simulink model "Arm_cobot"  (Simulink 8.3)
settings: Solver=ode1  StartTime=0.0  StopTime=inf  FixedStep=TA  RelTol=1e-3
PreLoadFcn:
  | startup
  | gui_starter
  | init_starter
PostLoadFcn:
  | init_check
InitFcn:
  | init_starter
undefined symbols (not defined in the file): alphaM, alphaT, Arm7ConLib, Arms2, baseOffset_x, baseOffset_y, baseOffset_z, betaM, betaT, cobotNa, cobotNb, D1, D2, D3, D4, D5, D6, D7, d_FTS_EE_L, d_FTS_EE_R, DD1, DD2, DD3, DD4, DD5, DD6, DD7, Do, Dp, EEL, EER, Fcal_L, Fcal_R, I1, I2, I3, I4, I5, I6, I7, IFL, IFR, impuls2rad_L, impuls2rad_R, Inert_L, Inert_R, KdC, KiC, Ko, Kp, KpC, LTool_L, LTool_R, mEE_L, mEE_R, Mo, Mp, P1, P2, P3 ... (+28)
libraries: sensoray x16, rtai_utilities x11, simulink x2, jr3lib x2, Interface x1
(part 1 of 3)
settings Model: Creator=mock  LastModifiedBy=wirnshofer  SimulationMode=external  ExtModeAutoUpdateStatusClock=off
settings DataIOCC: LimitDataPoints=off  SaveFormat=Structure
settings OptimizationCC: BlockReduction=off  BooleanDataType=off  ExpressionDepthLimit=2147483647  InitFltsAndDblsToZero=on
settings DebuggingCC: AlgebraicLoopMsg=none  SaveWithParameterizedLinksMsg=none  SignalResolutionControl=TryResolveAllWithWarning  SolverPrmCheckMsg=none  MultiTaskDSMMsg=warning  MultiTaskCondExecSysMsg=none  FcnCallInpInsideContextMsg=UseLocalSettings  UnconnectedInputMsg=none  UnconnectedOutputMsg=none  UnconnectedLineMsg=none  StrictBusMsg=None
settings HardwareCC: TargetHWDeviceType=32-bit Generic
settings SFSimCC: SimParseCustomCode=off
settings RTWCC: SystemTargetFile=prt.tlc  TemplateMakefile=prt.tmf  Description=Linux PREEMPT_RT Real-Time Target  ProcessScript=prt_make_rtw_hook  CustomLibrary=../../../../lib/libKinematicTypes.a ../../../../lib/libManipulation.a ../../../../lib/libkogmo_rtdb.a  IncludeERTFirstTime=on
settings RTWCC: CustomInclude=|
  | ../sfunctions/COMMON/InterfaceNew
  | ../sfunctions/COMMON/CollisionDetection
  | ../sfunctions/COMMON/PoseInterpolationNew
  | ../sfunctions/COMMON/PoseSpeedInterpolation
  | ../sfunctions/COMMON/Switching
  | ../sfunctions/COMMON/Helper
  | ../sfunctions/COMMON/Information
  | ../library/Animation
  | ../../../arch/rtdbobjects
  | ../../../arch
  | ../../../../opt/kogmo-rtdb/include
settings RTWCC: CustomSource=|
  | constant_information.cpp
  | ArmInterfaceNew.cpp
  | SwitchingX.cpp
  | Command_Classifier.cpp
  | PoseInterpolation_Code.cpp
  | PoseSpeedInterpolation_Code.cpp
  | armCDInterface.cpp
settings STFCustomTargetCC: TargetLangStandard=C99 (ISO)  CodeReplacementLibrary=GNU99 (GNU)  ModelReferenceCompliant=off  GeneratePreprocessorConditionals=Disable all  MatFileLogging=on  CPPClassGenCompliant=on  SystemTargetFile=prt.tlc
settings GRTTargetCC: TargetLangStandard=C99 (ISO)  CodeReplacementLibrary=GNU99 (GNU)  ModelReferenceCompliant=off  ParMdlRefBuildCompliant=off  CompOptLevelCompliant=off  ConcurrentExecutionCompliant=off  ExtModeMexArgs='cobot2a'

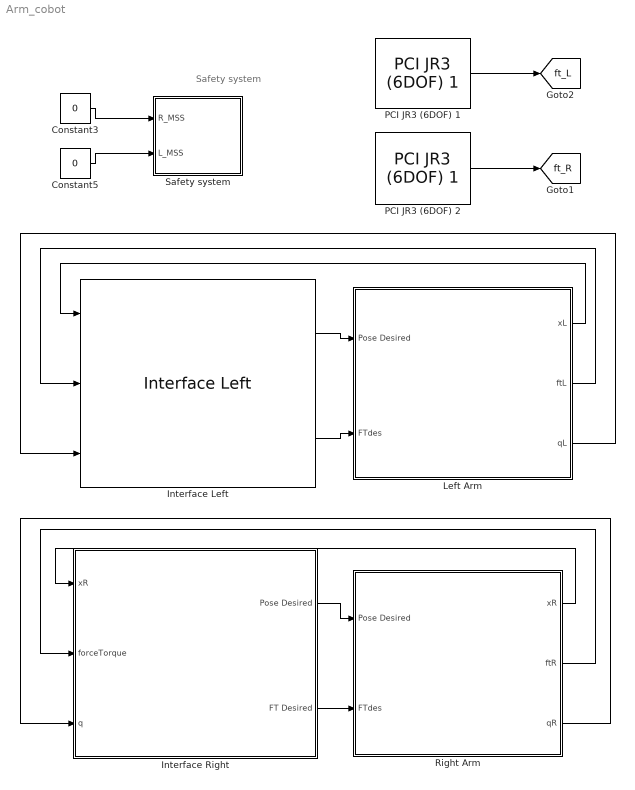
== system Arm_cobot ==
  note: Safety system
  Constant3 : Constant  Value=0
  Constant5 : Constant  Value=0
  Interface Left : Interface/Interface Left  SystemSampleTime=-1
  Interface Right : Subsystem  AncestorBlock=Interface/Interface Right  mask(Interface right){}
      settings: CopyFcn=inital_sources
      mask Display:
      | image(imread('Cobot_right.png'))
      | color('blue');
      | port_label('input',1, 'xR')
      | port_label('input',2, 'forceTorque')
      | port_label('input',3, 'q')
      | 
      | port_label('output',1, 'Pose Desired')
      | port_label('output',2, 'FT Desired')
  Left Arm : Subsystem  Priority=1
  PCI JR3 (6DOF) 1 : jr3lib/PCI JR3 (6DOF) 1  bd_number=0  filter_nr=1  sampletime=simget(bdroot,'FixedStep')  begin_reset=off
  PCI JR3 (6DOF) 2 : jr3lib/PCI JR3 (6DOF) 1  bd_number=1  filter_nr=1  sampletime=simget(bdroot,'FixedStep')  begin_reset=off
  Right Arm : Subsystem  Priority=1
  Safety system : Subsystem
      mask Display: image(imread('RTAIstop.bmp'))
  tag scope: ft_L=global, ft_R=global
  wires:
  Left Arm/2(ftL) -> Interface Left/2
  Right Arm/2(ftR) -> Interface Right/2(forceTorque)
  PCI JR3 (6DOF) 1/1 -> [ft_L]
  Constant3/1 -> Safety system/1(R_MSS)
  Constant5/1 -> Safety system/2(L_MSS)
  PCI JR3 (6DOF) 2/1 -> [ft_R]
  Interface Left/1 -> Left Arm/1(Pose Desired)
  Interface Right/1(Pose Desired) -> Right Arm/1(Pose Desired)
  Interface Left/2 -> Left Arm/2(FTdes)
  Left Arm/1(xL) -> Interface Left/1
  Left Arm/3(qL) -> Interface Left/3
  Interface Right/2(FT Desired) -> Right Arm/2(FTdes)
  Right Arm/1(xR) -> Interface Right/1(xR)
  Right Arm/3(qR) -> Interface Right/3(q)

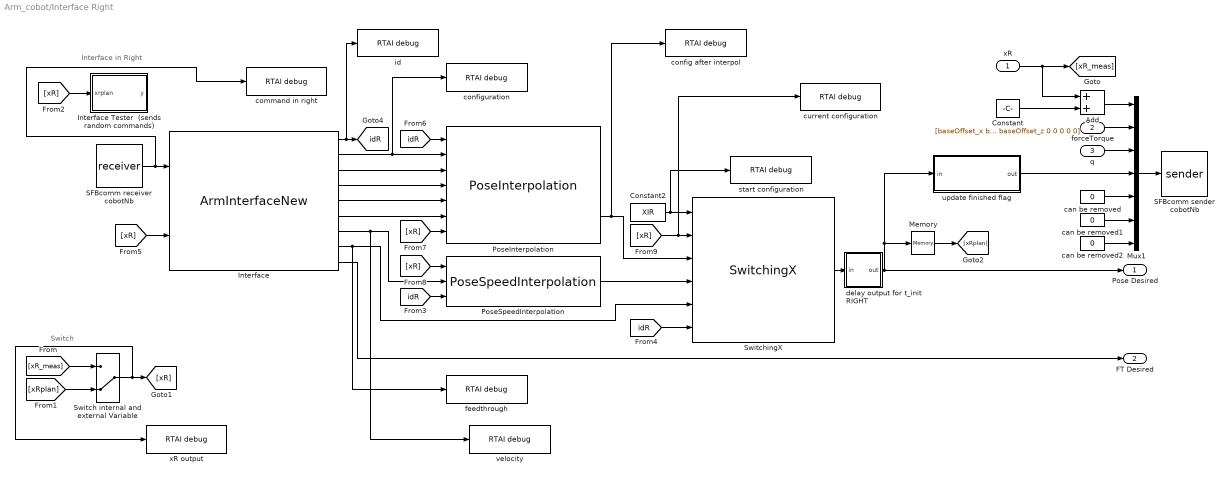
== system Arm_cobot/Interface Right ==
  note: Switch
  note: Interface in Right
  xR : Inport
  forceTorque : Inport  Port=2
  q : Inport  Port=3
  Add : Sum
  Constant : Constant  Value=[baseOffset_x baseOffset_y baseOffset_z 0 0 0 0 0]
  Constant2 : Constant  Value=XIR
  Interface : S-Function  FunctionName=ArmInterfaceNew  Parameters=xoffset,yoffset,zoffset  EnableBusSupport=off  mask{xoffset=baseOffset_x, yoffset=baseOffset_y, zoffset=baseOffset_z}
      mask prompts: xoffset "Base X Offset"; yoffset "Base Y Offset"; zoffset "Base Z Offset"
      mask Display:
      | port_label('input',1,'Command In')
      | port_label('input',2,'Configuration Current')
      | 
      | port_label('output',1,'CmdId')
      | port_label('output',2,'Configuration')
      | port_label('output',3,'Flags (replan/via)')
      | port_label('output',4,'Control Flow (count/total)')
      | port_label('output',5,'Time')
      | port_label('output',6,'Derivatives')
      | port_label('output',7,'Configuration Velocity')
      | port_label('output',8,'Feedthrough')
      | port_label('output',9,'FT')
  Interface Tester  (sends random commands) : MATLAB Function  TreatAsAtomicUnit=on
  Memory : Memory
  Mux1 : Mux  Inputs=7
  PoseInterpolation : S-Function  FunctionName=PoseInterpolation  EnableBusSupport=off
      mask Display:
      | port_label('input',1,'CmdId')
      | port_label('input',2,'Goal Configuration')
      | port_label('input',3,'Flags')
      | port_label('input',4,'Control Flow')
      | port_label('input',5,'Time')
      | port_label('input',6,'Derivatives')
      | port_label('input',7,'Current Configuration')
      | 
      | port_label('output',1,'Finish')
      | port_label('output',2,'Configuration')
  PoseSpeedInterpolation : S-Function  FunctionName=PoseSpeedInterpolation  EnableBusSupport=off
      mask Display:
      | port_label('input',1,'Current Configuration')
      | port_label('input',2,'Goal Configuration Speed')
      | port_label('input',3,'CmdId')
      | 
      | port_label('output',1,'Configuration')
  SFBcomm receiver cobotNb : S-Function  FunctionName=receiver  Parameters=localPort streamID remoteSettings portNames portWidths sampleTime outputLatency outputIdleTime connectTimeout  EnableBusSupport=off  mask(SFBcomm){localPort=8565, streamID=2, remoteSettings=[cobotNb ':8566'], portNames=A, portWidths=23, outputLatency=off, outputIdleTime=off, connectTimeout=200, sampleTime=TA}
      mask prompts: localPort "Local Port"; streamID "Stream ID"; remoteSettings "Remote Settings"; portNames "Port Names"; portWidths "Port Widths"; outputLatency "Output Latency"; outputIdleTime "Output Idle Time"; connectTimeout "Connect Timeout (in ms)"; sampleTime "Sample Time (-1 for inherited):"
      mask help: Receives data via SFB comm
      mask init:
      | idx=[0 strfind(portNames,' ') length(portNames)];
      | ddt=strfind(outputLatency,'on');
      | dit=strfind(outputIdleTime,'on');
      | 
      | for i=1:17
      |  if(i<length(idx))
      |   portnumber(i)=i;
      |   label{i}=portNames(idx(i)+1:idx(i+1));
      |  elseif((i==length(idx))&&(length(ddt)>0))
      |   portnumber(i)=i;
      |   label{i}='dt';
      |  elseif((i==length(idx))&&(length(dit)>0))
      |   portnumber(i)=i;
      |   label{i}='it';
      |  elseif((i==length(idx)+1)&&(length(ddt)>0)&&(length(dit)>0))
      |   portnumber(i)=i;
      |   label{i}='it';
      |  else
      |   portnumber(i)=1;
      |   label{i}=label{1};
      |  end
      | end
      mask Display:
      | image(imread('sfbcomm1.bmp'))
      | 
      | port_label('output',portnumber( 1),label{ 1})
      | port_label('output',portnumber( 2),label{ 2})
      | port_label('output',portnumber( 3),label{ 3})
      | port_label('output',portnumber( 4),label{ 4})
      | port_label('output',portnumber( 5),label{ 5})
      | port_label('output',portnumber( 6),label{ 6})
      | port_label('output',portnumber( 7),label{ 7})
      | port_label('output',portnumber( 8),label{ 8})
      | port_label('output',portnumber( 9),label{ 9})
      | port_label('output',portnumber(10),label{10})
      | port_label('output',portnumber(11),label{11})
      | port_label('output',portnumber(12),label{12})
      | port_label('output',portnumber(13),label{13})
      | port_label('output',portnumber(14),label{14})
      | port_label('output',portnumber(15),label{15})
      | port_label('output',portnumber(16),label{16})
      | port_label('output',portnumber(17),label{17})
  SFBcomm sender cobotNb : S-Function  FunctionName=sender  Parameters=localPort streamID remoteSettings portNames sampleTime connectTimeout  EnableBusSupport=off  mask(SFBcomm){localPort=8665, streamID=3, remoteSettings=[cobotNb ':8666'], portNames=A, connectTimeout=200, sampleTime=-1}
      mask prompts: localPort "Local Port"; streamID "Stream ID"; remoteSettings "Remote Settings"; portNames "Port Names"; connectTimeout "Connect Timeout (in ms)"; sampleTime "Sample time (-1 for inherited):"
      mask help: Sends data via SFB comm
      mask init:
      | idx=[0 strfind(portNames,' ') length(portNames)];
      | 
      | for i=1:16
      |  if(i<length(idx))
      |   portnumber(i)=i;
      |   label{i}=portNames(idx(i)+1:idx(i+1));
      |  else
      |   portnumber(i)=1;
      |   label{i}=label{1};
      |  end
      | end
      mask Display:
      | image(imread('sfbcomm1.bmp'))
      | port_label('input',portnumber( 1),label{ 1})
      | port_label('input',portnumber( 2),label{ 2})
      | port_label('input',portnumber( 3),label{ 3})
      | port_label('input',portnumber( 4),label{ 4})
      | port_label('input',portnumber( 5),label{ 5})
      | port_label('input',portnumber( 6),label{ 6})
      | port_label('input',portnumber( 7),label{ 7})
      | port_label('input',portnumber( 8),label{ 8})
      | port_label('input',portnumber( 9),label{ 9})
      | port_label('input',portnumber(10),label{10})
      | port_label('input',portnumber(11),label{11})
      | port_label('input',portnumber(12),label{12})
      | port_label('input',portnumber(13),label{13})
      | port_label('input',portnumber(14),label{14})
      | port_label('input',portnumber(15),label{15})
      | port_label('input',portnumber(16),label{16})
  Switch internal and external Variable : ManualSwitch  CurrentSetting=0
  SwitchingX : S-Function  FunctionName=SwitchingX  EnableBusSupport=off
      mask Display:
      | port_label('input',1,'Start Configuration')
      | port_label('input',2,'Current Configuration')
      | port_label('input',3,'Config from PoseInter')
      | port_label('input',4,'Config from SpeedInter')
      | port_label('input',5,'Config from Feedtrough')
      | port_label('input',6,'CmdId')
      | 
      | port_label('output',1,'Configuration')
  can be removed : Constant  Value=0
  can be removed1 : Constant  Value=0
  can be removed2 : Constant  Value=0
  command in right : rtai_utilities/RTAI debug  rate=1
  config after interpol : rtai_utilities/RTAI debug  rate=1
  configuration : rtai_utilities/RTAI debug  rate=1
  current configuration : rtai_utilities/RTAI debug  rate=1
  delay output for t_init RIGHT : Subsystem
  feedthrough : rtai_utilities/RTAI debug  rate=1
  id : rtai_utilities/RTAI debug  rate=1
  start configuration : rtai_utilities/RTAI debug  rate=1
  update finished flag : MATLAB Function  TreatAsAtomicUnit=on
  velocity : rtai_utilities/RTAI debug  rate=1
  xR output : rtai_utilities/RTAI debug  rate=1
  Pose Desired : Outport
  FT Desired : Outport  Port=2
  tag scope: idR=global
  wires:
  Switch internal and external Variable/1 -> xR output/1, [xR]
  [xRplan] -> Switch internal and external Variable/2
  Memory/1 -> [xRplan]
  [xR_meas] -> Switch internal and external Variable/1
  xR/1 -> [xR_meas], Add/1
  Constant2/1 -> start configuration/1, SwitchingX/1
  [xR] -> current configuration/1, SwitchingX/2
  PoseInterpolation/2 -> config after interpol/1, SwitchingX/3
  PoseSpeedInterpolation/1 -> SwitchingX/4
  Interface/8 -> feedthrough/1, SwitchingX/5
  [idR] -> SwitchingX/6
  [xR] -> Interface/2
  [xR] -> PoseSpeedInterpolation/1
  [xR] -> PoseInterpolation/7
  SFBcomm receiver cobotNb/1 -> command in right/1, Interface/1
  [xR] -> Interface Tester  (sends random commands)/1(xrplan)
  Interface/9 -> FT Desired/1
  update finished flag/1(out) -> Mux1/4
  [idR] -> PoseInterpolation/1
  Interface/6 -> PoseInterpolation/6
  Interface/5 -> PoseInterpolation/5
  delay output for t_init RIGHT/1(out) -> Memory/1, update finished flag/1(in), Pose Desired/1
  Interface/7 -> velocity/1, PoseSpeedInterpolation/2
  [idR] -> PoseSpeedInterpolation/3
  Interface/1 -> id/1, [idR]
  SwitchingX/1 -> delay output for t_init RIGHT/1(in)
  can be removed2/1 -> Mux1/7
  can be removed1/1 -> Mux1/6
  can be removed/1 -> Mux1/5
  Constant/1 -> Add/2
  Add/1 -> Mux1/1
  Mux1/1 -> SFBcomm sender cobotNb/1
  q/1 -> Mux1/3
  forceTorque/1 -> Mux1/2
  Interface/4 -> PoseInterpolation/4
  Interface/3 -> PoseInterpolation/3
  Interface/2 -> configuration/1, PoseInterpolation/2

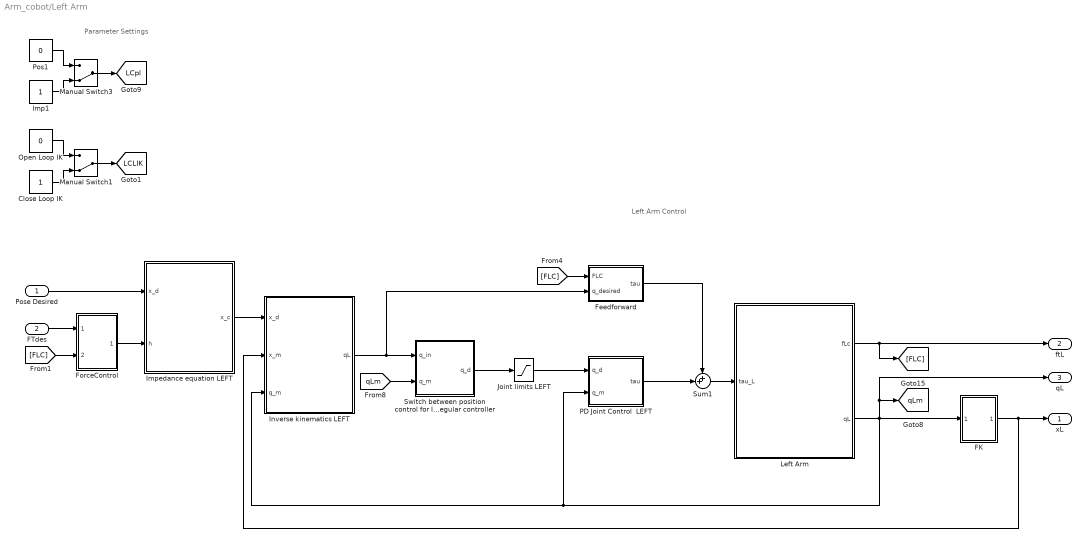
== system Arm_cobot/Left Arm ==
  note: Parameter Settings
  note: Left Arm Control
  Pose Desired : Inport
  FTdes : Inport  Port=2
  Close Loop IK : Constant
  FK : Subsystem
  Feedforward : Subsystem
  ForceControl : Subsystem
  Imp1 : Constant
  Impedance equation LEFT : Subsystem
  Inverse kinematics LEFT : Subsystem
  Joint limits LEFT : Saturate  UpperLimit=q_maxL  LowerLimit=q_minL
  Left Arm : Subsystem
  Manual Switch1 : ManualSwitch  Priority=1  CurrentSetting=0
  Manual Switch3 : ManualSwitch  Priority=1  CurrentSetting=0
  Open Loop IK : Constant  Value=0
  PD Joint Control  LEFT : Subsystem  AncestorBlock=Arm7lib/PD Joint
  Pos1 : Constant  Value=0
  Sum1 : Sum  Inputs=++|
  Switch between position control for Init position and regular controller : Subsystem
  xL : Outport
  ftL : Outport  Port=2
  qL : Outport  Port=3
  tag scope: LCLIK=global, LCpl=global, qLm=global
  wires:
  Left Arm/2(qL) -> FK/1(q_m), PD Joint Control  LEFT/2(q_m), Inverse kinematics LEFT/3(q_m), qL/1, [qLm]
  Left Arm/1(fLc) -> ftL/1, [FLC]
  [qLm] -> Switch between position control for Init position and regular controller/2(q_m)
  Joint limits LEFT/1 -> PD Joint Control  LEFT/1(q_d)
  Imp1/1 -> Manual Switch3/2
  Pos1/1 -> Manual Switch3/1
  Manual Switch3/1 -> [LCpl]
  Switch between position control for Init position and regular controller/1(q_d) -> Joint limits LEFT/1
  Pose Desired/1 -> Impedance equation LEFT/1(x_d)
  FK/1(pose) -> xL/1, Inverse kinematics LEFT/2(x_m)
  Inverse kinematics LEFT/1(qL) -> Switch between position control for Init position and regular controller/1(q_in), Feedforward/2(q_desired)
  Close Loop IK/1 -> Manual Switch1/2
  Open Loop IK/1 -> Manual Switch1/1
  Manual Switch1/1 -> [LCLIK]
  ForceControl/1(Out1) -> Impedance equation LEFT/2(h)
  [FLC] -> ForceControl/2(FTmesL)
  FTdes/1 -> ForceControl/1(FTdesLeft)
  Sum1/1 -> Left Arm/1(tau_L)
  PD Joint Control  LEFT/1(tau) -> Sum1/2
  Impedance equation LEFT/1(x_c) -> Inverse kinematics LEFT/1(x_d)
  [FLC] -> Feedforward/1(FLC)
  Feedforward/1(tau) -> Sum1/1

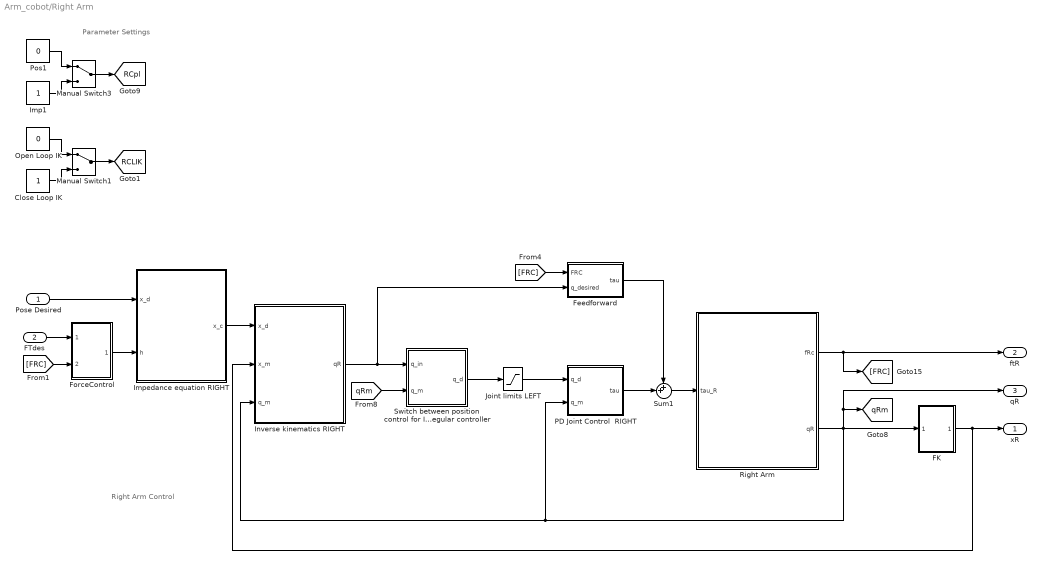
== system Arm_cobot/Right Arm ==
  note: Parameter Settings
  note: Right Arm Control
  Pose Desired : Inport
  FTdes : Inport  Port=2
  Close Loop IK : Constant
  FK : Subsystem
  Feedforward : Subsystem
  ForceControl : Subsystem
  Imp1 : Constant
  Impedance equation RIGHT : Subsystem
  Inverse kinematics RIGHT : Subsystem
  Joint limits LEFT : Saturate  UpperLimit=q_maxR  LowerLimit=q_minR
  Manual Switch1 : ManualSwitch
  Manual Switch3 : ManualSwitch
  Open Loop IK : Constant  Value=0
  PD Joint Control  RIGHT : Subsystem  AncestorBlock=Arm7lib/PD Joint
  Pos1 : Constant  Value=0
  Right Arm : Subsystem
  Sum1 : Sum  Inputs=++|
  Switch between position control for Init position and regular controller : Subsystem
  xR : Outport
  ftR : Outport  Port=2
  qR : Outport  Port=3
  tag scope: RCLIK=global, RCpl=global, qRm=global
  wires:
  Right Arm/2(qR) -> FK/1(q_m), PD Joint Control  RIGHT/2(q_m), Inverse kinematics RIGHT/3(q_m), qR/1, [qRm]
  Right Arm/1(fRc) -> ftR/1, [FRC]
  [qRm] -> Switch between position control for Init position and regular controller/2(q_m)
  Joint limits LEFT/1 -> PD Joint Control  RIGHT/1(q_d)
  Imp1/1 -> Manual Switch3/2
  Pos1/1 -> Manual Switch3/1
  Manual Switch3/1 -> [RCpl]
  Switch between position control for Init position and regular controller/1(q_d) -> Joint limits LEFT/1
  Sum1/1 -> Right Arm/1(tau_R)
  Pose Desired/1 -> Impedance equation RIGHT/1(x_d)
  FK/1(pose) -> xR/1, Inverse kinematics RIGHT/2(x_m)
  Inverse kinematics RIGHT/1(qR) -> Switch between position control for Init position and regular controller/1(q_in), Feedforward/2(q_desired)
  Close Loop IK/1 -> Manual Switch1/2
  Open Loop IK/1 -> Manual Switch1/1
  Manual Switch1/1 -> [RCLIK]
  [FRC] -> Feedforward/1(FRC)
  FTdes/1 -> ForceControl/1(FTdesRight)
  [FRC] -> ForceControl/2(FTmesR)
  ForceControl/1(Out1) -> Impedance equation RIGHT/2(h)
  Impedance equation RIGHT/1(x_c) -> Inverse kinematics RIGHT/1(x_d)
  PD Joint Control  RIGHT/1(tau) -> Sum1/2
  Feedforward/1(tau) -> Sum1/1

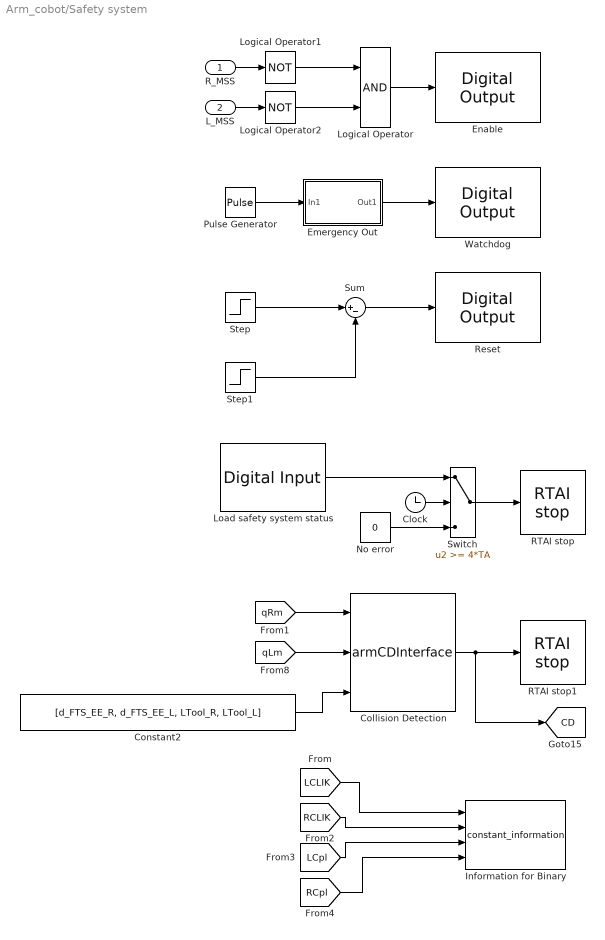
== system Arm_cobot/Safety system ==
  R_MSS : Inport
  L_MSS : Inport  Port=2
  Clock : Clock
  Collision Detection : S-Function  FunctionName=armCDInterface  EnableBusSupport=off
  Constant2 : Constant  Value=[d_FTS_EE_R, d_FTS_EE_L, LTool_R, LTool_L]
  Emergency Out : Subsystem
  Enable : sensoray/Digital Output  BoardNumber=0  Channels=27  InitialOutputs=0  FinalOutputs=0  SampleTime=-1
  Information for Binary : S-Function  Priority=2  FunctionName=constant_information  Parameters="cobotNa, EEL, EER,  get_param('Arm_cobot/Interface Left/Switch internal and external Variable', 'sw'), get_param('Arm_cobot/Interface Right/Switch internal and external Variable', 'sw')"  EnableBusSupport=off
  Load safety system status : sensoray/Digital Input  BoardNumber=0  Channels=25  SampleTime=simget(bdroot,'FixedStep')
  Logical Operator : Logic  AllPortsSameDT=off
  Logical Operator1 : Logic  Operator=NOT  AllPortsSameDT=off  OutDataTypeStr=boolean
  Logical Operator2 : Logic  Operator=NOT  AllPortsSameDT=off  OutDataTypeStr=boolean
  No error : Constant  Value=0
  Pulse Generator : DiscretePulseGenerator  PulseType=Time based  Period=2*TA  PulseWidth=50
  RTAI stop : rtai_utilities/RTAI stop
  RTAI stop1 : rtai_utilities/RTAI stop
  Reset : sensoray/Digital Output  BoardNumber=0  Channels=24  InitialOutputs=0  FinalOutputs=0  SampleTime=-1
  Step : Step  Time=0
  Step1 : Step  Time=2*TA
  Sum : Sum  Inputs=|+-  SaturateOnIntegerOverflow=on  InputSameDT=on  OutDataTypeStr=Inherit: Same as first input
  Switch : Switch  Threshold=4*TA  SaturateOnIntegerOverflow=on  InputSameDT=on
  Watchdog : sensoray/Digital Output  BoardNumber=0  Channels=26  InitialOutputs=0  FinalOutputs=0  SampleTime=-1
  tag scope: CD=global
  wires:
  Pulse Generator/1 -> Emergency Out/1(In1)
  Step/1 -> Sum/1
  Sum/1 -> Reset/1
  Step1/1 -> Sum/2
  Logical Operator/1 -> Enable/1
  R_MSS/1 -> Logical Operator1/1
  L_MSS/1 -> Logical Operator2/1
  Logical Operator1/1 -> Logical Operator/1
  Logical Operator2/1 -> Logical Operator/2
  Switch/1 -> RTAI stop/1
  Clock/1 -> Switch/2
  Load safety system status/1 -> Switch/1
  No error/1 -> Switch/3
  Collision Detection/1 -> RTAI stop1/1, [CD]
  [qLm] -> Collision Detection/2
  [qRm] -> Collision Detection/1
  Constant2/1 -> Collision Detection/3
  Emergency Out/1(Out1) -> Watchdog/1
  [LCLIK] -> Information for Binary/1
  [LCpl] -> Information for Binary/3
  [RCpl] -> Information for Binary/4
  [RCLIK] -> Information for Binary/2

== system Arm_cobot/Interface Right/delay output for t_init RIGHT ==
  in : Inport
  Clock : Clock
  Constant1 : Constant  Value=XIR
  Switch2 : Switch  Threshold=t_init  SaturateOnIntegerOverflow=on  InputSameDT=on
  out : Outport
  wires:
  Switch2/1 -> out/1
  in/1 -> Switch2/1
  Constant1/1 -> Switch2/3
  Clock/1 -> Switch2/2

== system Arm_cobot/Left Arm/FK ==
  q_m : Inport
  Constant1 : Constant  Value=LTool_L
  Demux : Demux  Outputs=[3 9 1]
  FK_L : S-Function  FunctionName=fk_l_S  EnableBusSupport=off
  Mux : Mux  Inputs=2
  Mux1 : Mux  Inputs=3
  Reshape : Reshape  OutputDimensionality=Customize  OutputDimensions=[3,3]
  S-Function1 : S-Function  FunctionName=rot2Q_S  EnableBusSupport=off
  pose : Outport
  wires:
  Constant1/1 -> Mux/1
  Mux/1 -> FK_L/1
  FK_L/1 -> Demux/1
  Demux/1 -> Mux1/1
  Demux/3 -> Mux1/3
  q_m/1 -> Mux/2
  Mux1/1 -> pose/1
  Reshape/1 -> S-Function1/1
  Demux/2 -> Reshape/1
  S-Function1/1 -> Mux1/2

== system Arm_cobot/Left Arm/Feedforward ==
  FLC : Inport
  q_desired : Inport  Port=2
  Constant1 : Constant  Value=[0 0 0 0 0 0]
  Constant2 : Constant  Value=[Inert_L, d_FTS_EE_L, mEE_L, p_EE_o_L]
  Demux : Demux  Outputs=[3,3]
  Derivative : Derivative
  Gain : Gain  Gain=-1
  Mux2 : Mux  Inputs=6
  S-Function : S-Function  FunctionName=dynmod_l_S  EnableBusSupport=off
  second  derivative : Subsystem  AncestorBlock=Arm7lib/PD Joint
  tau : Outport
  wires:
  q_desired/1 -> Mux2/3, Derivative/1, second  derivative/1(q)
  Mux2/1 -> S-Function/1
  S-Function/1 -> tau/1
  Constant2/1 -> Mux2/1
  Derivative/1 -> Mux2/5
  Demux/1 -> Mux2/2
  Demux/2 -> Mux2/4
  Gain/1 -> Demux/1
  Constant1/1 -> Gain/1
  second  derivative/1(qDotDot) -> Mux2/6

== system Arm_cobot/Left Arm/ForceControl ==
  FTdesLeft : Inport
  FTmesL : Inport  Port=2
  Abs : Abs
  Subsystem : Subsystem  mask{PF=PFL, IF=IFL, SF=SFL}
      mask prompts: PF "Proportional Gain"; IF "Integral Gain"; SF "Saturation"
      mask Display: disp('PI6')
  Sum : Sum  Inputs=|++
  Sum of Elements : Sum  Inputs=+
  Switch : Switch  Criteria=u2 ~= 0  Threshold=0.5
  lowpass : Subsystem
  Out1 : Outport
  wires:
  Sum/1 -> Subsystem/1(In1)
  Subsystem/1(Out1) -> Switch/1
  FTdesLeft/1 -> Sum/2, Abs/1
  Abs/1 -> Sum of Elements/1
  Sum of Elements/1 -> Subsystem/2(reset), Switch/2
  FTmesL/1 -> lowpass/1(fLc), Switch/3
  Switch/1 -> Out1/1
  lowpass/1(smoothed) -> Sum/1

== system Arm_cobot/Left Arm/Impedance equation LEFT ==
  x_d : Inport
  h : Inport  Port=2
  Constant1 : Constant  Value=zeros(1,7)
  Impedance  Equation : Subsystem  AncestorBlock="Arm7ConLib/Impedance  Equation"  mask{M_p=Mp, D_p=Dp, K_p=Kp, M_o=Mo, D_o=Do, K_o=Ko}
      mask prompts: M_p "Virtual mass (Translational)"; D_p "Damping matrix (translational)"; K_p "Stiffness matrix (translational)"; M_o "Virtual mass (rotational)"; D_o "Damping matrix (rotational)"; K_o "Stiffness matrix (rotational)"
  Switch : Switch  Threshold=0.5
  x_c : Outport
  wires:
  Constant1/1 -> Impedance  Equation/3(ddx_d), Impedance  Equation/2(dx_d)
  h/1 -> Impedance  Equation/4(h)
  x_d/1 -> Impedance  Equation/1(x_d), Switch/3
  Switch/1 -> x_c/1
  [LCpl] -> Switch/2
  Impedance  Equation/1(x_c) -> Switch/1

== system Arm_cobot/Left Arm/Inverse kinematics LEFT ==
  x_d : Inport
  x_m : Inport  Port=2
  q_m : Inport  Port=3
  IK_L weighted damped least square : Subsystem
  Pos1 : Constant  Value=zeros(7,1)
  Switch : Switch  Threshold=0.5
  pose error in task space : Subsystem
  qL : Outport
  wires:
  x_d/1 -> IK_L weighted damped least square/1(XL), pose error in task space/1(x_d)
  x_m/1 -> pose error in task space/2(x_m)
  IK_L weighted damped least square/1(q_damp) -> qL/1, IK_L weighted damped least square/2(qL)
  q_m/1 -> pose error in task space/3(qL)
  [LCLIK] -> Switch/2
  Switch/1 -> IK_L weighted damped least square/3(X_error)
  pose error in task space/1(X_error) -> Switch/1
  Pos1/1 -> Switch/3

== system Arm_cobot/Left Arm/Left Arm ==
  tau_L : Inport
  Arms : Subsystem  AncestorBlock=Arm7ConLib/Arms2
  fLc : Outport
  qL : Outport  Port=2
  wires:
  Arms/1(q _L) -> qL/1
  Arms/3(fLc) -> fLc/1
  tau_L/1 -> Arms/1(tau_L)

== system Arm_cobot/Left Arm/PD Joint Control  LEFT ==
  q_d : Inport
  q_m : Inport  Port=2
  PID Digital Derivative1 : Subsystem  mask(7 DOF PID Controller){P=[P1 P2 P3 P4 P5 P6 P7], I=[I1 I2 I3 I4 I5 I6 I7], D=[D1 D2 D3 D4 D5 D6 D7], N=[DD1 DD2 DD3 DD4 DD5 DD6 DD7]}
      mask prompts: P "Proportional:"; I "Integral"; D "Derivative:"; N "Derivative Divisor:"
      mask Display: disp('PID7')
  Sum1 : Sum  Inputs=-+|  SaturateOnIntegerOverflow=on  InputSameDT=on  OutDataTypeStr=Inherit: Same as first input
  tau : Outport
  wires:
  q_d/1 -> Sum1/2
  q_m/1 -> Sum1/1
  Sum1/1 -> PID Digital Derivative1/1(In1)
  PID Digital Derivative1/1(Out1) -> tau/1

== system Arm_cobot/Left Arm/Switch between position control for Init position and regular controller ==
  q_in : Inport
  q_m : Inport  Port=2
  BackToInit1 : Subsystem
  Clock : Clock
  Switch2 : Switch  Threshold=t_init  SaturateOnIntegerOverflow=on  InputSameDT=on
  q_d : Outport
  wires:
  q_in/1 -> Switch2/1
  Clock/1 -> Switch2/2
  BackToInit1/1(q [rad]) -> Switch2/3
  q_m/1 -> BackToInit1/1(JointAngles [rad])
  Switch2/1 -> q_d/1

== system Arm_cobot/Right Arm/FK ==
  q_m : Inport
  Constant1 : Constant  Value=LTool_R
  Demux : Demux  Outputs=[3 9 1]
  FK_R : S-Function  FunctionName=fk_r_S  EnableBusSupport=off
  Mux : Mux  Inputs=2
  Mux1 : Mux  Inputs=3
  Reshape : Reshape  OutputDimensionality=Customize  OutputDimensions=[3,3]
  S-Function1 : S-Function  FunctionName=rot2Q_S  EnableBusSupport=off
  pose : Outport
  wires:
  Constant1/1 -> Mux/1
  Mux/1 -> FK_R/1
  FK_R/1 -> Demux/1
  Demux/1 -> Mux1/1
  Demux/3 -> Mux1/3
  q_m/1 -> Mux/2
  Mux1/1 -> pose/1
  Reshape/1 -> S-Function1/1
  Demux/2 -> Reshape/1
  S-Function1/1 -> Mux1/2

== system Arm_cobot/Right Arm/Feedforward ==
  FRC : Inport
  q_desired : Inport  Port=2
  Constant1 : Constant  Value=[0 0 0 0 0 0]
  Constant2 : Constant  Value=[Inert_R, d_FTS_EE_R, mEE_R, p_EE_o_R]
  Demux : Demux  Outputs=[3,3]
  Derivative : Derivative
  Gain : Gain  Gain=-1
  Mux2 : Mux  Inputs=6
  S-Function : S-Function  FunctionName=dynmod_r_S  EnableBusSupport=off
  second  derivative : Subsystem  AncestorBlock=Arm7lib/PD Joint
  tau : Outport
  wires:
  q_desired/1 -> Mux2/3, Derivative/1, second  derivative/1(q)
  Mux2/1 -> S-Function/1
  S-Function/1 -> tau/1
  Constant2/1 -> Mux2/1
  Derivative/1 -> Mux2/5
  Demux/1 -> Mux2/2
  Demux/2 -> Mux2/4
  Gain/1 -> Demux/1
  Constant1/1 -> Gain/1
  second  derivative/1(qDotDot) -> Mux2/6

== system Arm_cobot/Right Arm/ForceControl ==
  FTdesRight : Inport
  FTmesR : Inport  Port=2
  Abs : Abs
  Subsystem : Subsystem  mask{PF=PFR, IF=IFR, SF=SFR}
      mask prompts: PF "Proportional Gain"; IF "Integral Gain"; SF "Saturation"
      mask Display: disp('PI6')
  Sum : Sum  Inputs=|++
  Sum of Elements : Sum  Inputs=+
  Switch : Switch  Criteria=u2 ~= 0  Threshold=0.5
  lowpass : Subsystem
  Out1 : Outport
  wires:
  Sum/1 -> Subsystem/1(In1)
  Subsystem/1(Out1) -> Switch/1
  FTdesRight/1 -> Sum/2, Abs/1
  Abs/1 -> Sum of Elements/1
  Sum of Elements/1 -> Subsystem/2(reset), Switch/2
  FTmesR/1 -> lowpass/1(fLc), Switch/3
  Switch/1 -> Out1/1
  lowpass/1(smoothed) -> Sum/1

== system Arm_cobot/Right Arm/Impedance equation RIGHT ==
  x_d : Inport
  h : Inport  Port=2
  Constant1 : Constant  Value=zeros(1,7)
  Impedance  Equation : Subsystem  AncestorBlock="Arm7ConLib/Impedance  Equation"  mask{M_p=Mp, D_p=Dp, K_p=Kp, M_o=Mo, D_o=Do, K_o=Ko}
      mask prompts: M_p "Virtual mass (Translational)"; D_p "Damping matrix (translational)"; K_p "Stiffness matrix (translational)"; M_o "Virtual mass (rotational)"; D_o "Damping matrix (rotational)"; K_o "Stiffness matrix (rotational)"
  Switch : Switch  Threshold=0.5
  x_c : Outport
  wires:
  Constant1/1 -> Impedance  Equation/3(ddx_d), Impedance  Equation/2(dx_d)
  Impedance  Equation/1(x_c) -> Switch/1
  h/1 -> Impedance  Equation/4(h)
  x_d/1 -> Impedance  Equation/1(x_d), Switch/3
  Switch/1 -> x_c/1
  [RCpl] -> Switch/2

== system Arm_cobot/Right Arm/Inverse kinematics RIGHT ==
  x_d : Inport
  x_m : Inport  Port=2
  q_m : Inport  Port=3
  IK_R weighted damped least square : Subsystem
  Switch : Switch  Threshold=0.5
  pose error in task space : Subsystem
  zeros : Constant  Value=zeros(7,1)
  qR : Outport
  wires:
  x_d/1 -> IK_R weighted damped least square/1(XR), pose error in task space/1(x_d)
  x_m/1 -> pose error in task space/2(x_m)
  IK_R weighted damped least square/1(q_damp) -> IK_R weighted damped least square/2(qR), qR/1
  q_m/1 -> pose error in task space/3(qR)
  [RCLIK] -> Switch/2
  Switch/1 -> IK_R weighted damped least square/3(X_error)
  pose error in task space/1(X_error) -> Switch/1
  zeros/1 -> Switch/3

== system Arm_cobot/Right Arm/PD Joint Control  RIGHT ==
  q_d : Inport
  q_m : Inport  Port=2
  PID Digital Derivative1 : Subsystem  mask(7 DOF PID Controller){P=[P1 P2 P3 P4 P5 P6 P7], I=[I1 I2 I3 I4 I5 I6 I7], D=[D1 D2 D3 D4 D5 D6 D7], N=[DD1 DD2 DD3 DD4 DD5 DD6 DD7]}
      mask prompts: P "Proportional:"; I "Integral"; D "Derivative:"; N "Derivative Divisor:"
      mask Display: disp('PID7')
  Sum1 : Sum  Inputs=-+|  SaturateOnIntegerOverflow=on  InputSameDT=on  OutDataTypeStr=Inherit: Same as first input
  tau : Outport
  wires:
  q_d/1 -> Sum1/2
  q_m/1 -> Sum1/1
  Sum1/1 -> PID Digital Derivative1/1(In1)
  PID Digital Derivative1/1(Out1) -> tau/1

== system Arm_cobot/Right Arm/Right Arm ==
  tau_R : Inport
  Arms : Subsystem  AncestorBlock=Arm7ConLib/Arms2
  fRc : Outport
  qR : Outport  Port=2
  wires:
  Arms/1(q _R) -> qR/1
  Arms/3(fRc) -> fRc/1
  tau_R/1 -> Arms/1(tau_R)

== system Arm_cobot/Right Arm/Switch between position control for Init position and regular controller ==
  q_in : Inport
  q_m : Inport  Port=2
  BackToInit1 : Subsystem
  Clock : Clock
  Switch2 : Switch  Threshold=t_init  SaturateOnIntegerOverflow=on  InputSameDT=on
  q_d : Outport
  wires:
  q_in/1 -> Switch2/1
  Clock/1 -> Switch2/2
  BackToInit1/1(q [rad]) -> Switch2/3
  q_m/1 -> BackToInit1/1(JointAngles [rad])
  Switch2/1 -> q_d/1

== system Arm_cobot/Safety system/Emergency Out ==
  In1 : Inport
  Fcn : Fcn  Expr=-u[1]+1
  Product : Product  RndMeth=Zero
  Out1 : Outport
  wires:
  [CD] -> Fcn/1
  In1/1 -> Product/2
  Product/1 -> Out1/1
  Fcn/1 -> Product/1

== system Arm_cobot/Left Arm/Feedforward/second  derivative ==
  q : Inport
  2ndDerivative3Points : MATLAB Function  TreatAsAtomicUnit=on
  Constant : Constant  Value=10*ones(1,7)
  Constant1 : Constant  Value=-10*ones(1,7)
  Memory : Memory
  Memory1 : Memory
  Rate Limiter Dynamic : simulink/Discontinuities/Rate Limiter Dynamic
  qDotDot : Outport
  wires:
  q/1 -> Memory/1, 2ndDerivative3Points/1(u0)
  Memory/1 -> Memory1/1, 2ndDerivative3Points/2(u1)
  Memory1/1 -> 2ndDerivative3Points/3(u2)
  Constant/1 -> Rate Limiter Dynamic/1
  Constant1/1 -> Rate Limiter Dynamic/3
  Rate Limiter Dynamic/1 -> qDotDot/1
  2ndDerivative3Points/1(y) -> Rate Limiter Dynamic/2

== system Arm_cobot/Left Arm/ForceControl/Subsystem ==
  In1 : Inport
  reset : Inport  Port=2
  Demux : Demux  Outputs=6
  Mux : Mux  Inputs=6
  PII : Subsystem  AncestorBlock=|  mask(PID(2) Controller){P=PF(1), I=IF(1), S=SF(1)}
      | Arm7lib/PID
      | Digital Derivative/PID +
      | digital Derivative2
      mask prompts: P "Proportional:"; I "Integral:"; S "Saturation:"
      mask help:
      | Enter Proportional(P), Integral(I), and Derivative(D) and divisor (N) terms.
      | P+I/s+Ds/(1/Ns+1)
      mask Help: This block implements a PID controller where parameters are entered for the Proportional, Integral and Derivative and divisor terms. Unmask this block to see how it works. The derivative term is implemented using an s/(s/N +1)  transfer function block. Making N large can create a "stiff" system.
      mask Display: disp('PI')
  PII1 : Subsystem  AncestorBlock=|  mask(PID(2) Controller){P=PF(2), I=IF(2), S=SF(2)}
      | Arm7lib/PID
      | Digital Derivative/PID +
      | digital Derivative2
      mask prompts: P "Proportional:"; I "Integral:"; S "Saturation:"
      mask help:
      | Enter Proportional(P), Integral(I), and Derivative(D) and divisor (N) terms.
      | P+I/s+Ds/(1/Ns+1)
      mask Help: This block implements a PID controller where parameters are entered for the Proportional, Integral and Derivative and divisor terms. Unmask this block to see how it works. The derivative term is implemented using an s/(s/N +1)  transfer function block. Making N large can create a "stiff" system.
      mask Display: disp('PI')
  PII2 : Subsystem  AncestorBlock=|  mask(PID(2) Controller){P=PF(3), I=IF(3), S=SF(3)}
      | Arm7lib/PID
      | Digital Derivative/PID +
      | digital Derivative2
      mask prompts: P "Proportional:"; I "Integral:"; S "Saturation:"
      mask help:
      | Enter Proportional(P), Integral(I), and Derivative(D) and divisor (N) terms.
      | P+I/s+Ds/(1/Ns+1)
      mask Help: This block implements a PID controller where parameters are entered for the Proportional, Integral and Derivative and divisor terms. Unmask this block to see how it works. The derivative term is implemented using an s/(s/N +1)  transfer function block. Making N large can create a "stiff" system.
      mask Display: disp('PI')
  PII3 : Subsystem  AncestorBlock=|  mask(PID(2) Controller){P=PF(4), I=IF(4), S=SF(4)}
      | Arm7lib/PID
      | Digital Derivative/PID +
      | digital Derivative2
      mask prompts: P "Proportional:"; I "Integral:"; S "Saturation:"
      mask help:
      | Enter Proportional(P), Integral(I), and Derivative(D) and divisor (N) terms.
      | P+I/s+Ds/(1/Ns+1)
      mask Help: This block implements a PID controller where parameters are entered for the Proportional, Integral and Derivative and divisor terms. Unmask this block to see how it works. The derivative term is implemented using an s/(s/N +1)  transfer function block. Making N large can create a "stiff" system.
      mask Display: disp('PI')
  PII4 : Subsystem  AncestorBlock=|  mask(PID(2) Controller){P=PF(5), I=IF(5), S=SF(5)}
      | Arm7lib/PID
      | Digital Derivative/PID +
      | digital Derivative2
      mask prompts: P "Proportional:"; I "Integral:"; S "Saturation:"
      mask help:
      | Enter Proportional(P), Integral(I), and Derivative(D) and divisor (N) terms.
      | P+I/s+Ds/(1/Ns+1)
      mask Help: This block implements a PID controller where parameters are entered for the Proportional, Integral and Derivative and divisor terms. Unmask this block to see how it works. The derivative term is implemented using an s/(s/N +1)  transfer function block. Making N large can create a "stiff" system.
      mask Display: disp('PI')
  PII5 : Subsystem  AncestorBlock=|  mask(PID(2) Controller){P=PF(6), I=IF(6), S=SF(6)}
      | Arm7lib/PID
      | Digital Derivative/PID +
      | digital Derivative2
      mask prompts: P "Proportional:"; I "Integral:"; S "Saturation:"
      mask help:
      | Enter Proportional(P), Integral(I), and Derivative(D) and divisor (N) terms.
      | P+I/s+Ds/(1/Ns+1)
      mask Help: This block implements a PID controller where parameters are entered for the Proportional, Integral and Derivative and divisor terms. Unmask this block to see how it works. The derivative term is implemented using an s/(s/N +1)  transfer function block. Making N large can create a "stiff" system.
      mask Display: disp('PI')
  Out1 : Outport
  wires:
  In1/1 -> Demux/1
  Demux/1 -> PII/1(In_1)
  Demux/2 -> PII1/1(In_1)
  Demux/3 -> PII2/1(In_1)
  Demux/5 -> PII4/1(In_1)
  PII/1(Out_1) -> Mux/1
  PII1/1(Out_1) -> Mux/2
  PII2/1(Out_1) -> Mux/3
  PII3/1(Out_1) -> Mux/4
  PII4/1(Out_1) -> Mux/5
  PII5/1(Out_1) -> Mux/6
  Mux/1 -> Out1/1
  Demux/6 -> PII5/1(In_1)
  reset/1 -> PII/2(reset), PII1/2(reset), PII2/2(reset), PII3/2(reset), PII5/2(reset), PII4/2(reset)
  Demux/4 -> PII3/1(In_1)

== system Arm_cobot/Left Arm/ForceControl/lowpass ==
  fLc : Inport
  Demux : Demux  Outputs=6
  Discrete Filter{,1..5} (6 alike) : DiscreteFilter  Numerator=[0.1 0.1 0.1 0.1 0.1 0.1 0.1 0.1 0.1 0.1]  Denominator=[1]
  Mux2 : Mux  Inputs=6
  Rate Transition3 : RateTransition  X0=-1
  smoothed : Outport
  wires:
  Discrete Filter/1 -> Mux2/1
  Demux/1 -> Discrete Filter/1
  Demux/2 -> Discrete Filter1/1
  Demux/3 -> Discrete Filter2/1
  Demux/4 -> Discrete Filter3/1
  Demux/5 -> Discrete Filter4/1
  Demux/6 -> Discrete Filter5/1
  Discrete Filter1/1 -> Mux2/2
  Discrete Filter3/1 -> Mux2/4
  Discrete Filter4/1 -> Mux2/5
  Discrete Filter5/1 -> Mux2/6
  Mux2/1 -> smoothed/1
  fLc/1 -> Rate Transition3/1
  Rate Transition3/1 -> Demux/1
  Discrete Filter2/1 -> Mux2/3

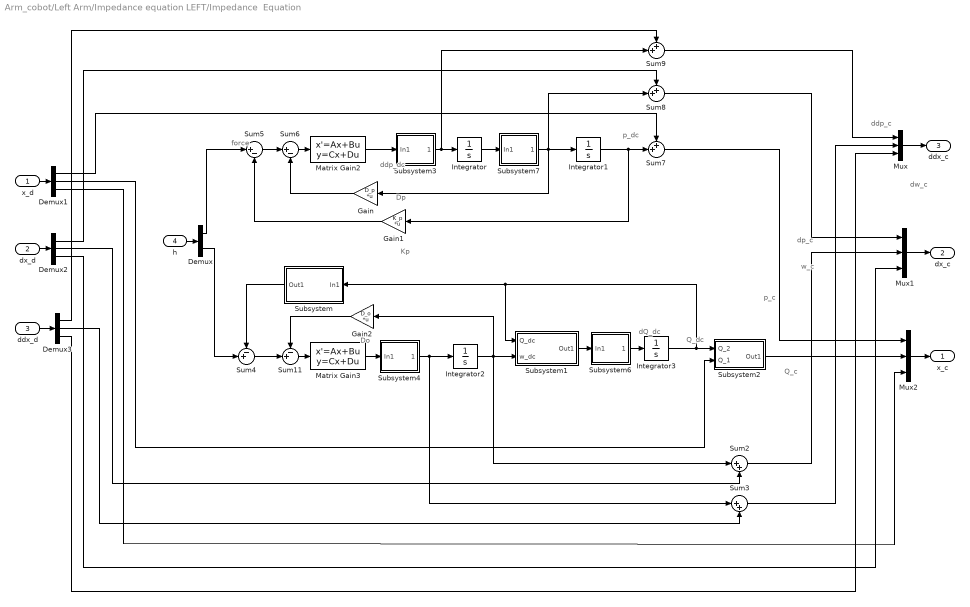
== system Arm_cobot/Left Arm/Impedance equation LEFT/Impedance  Equation ==
  note: Do
  note: Dp
  note: Kp
  note: p_dc
  note: ddp_dc
  note: force
  note: p_c
  note: dp_c
  note: ddp_c
  note: dQ_dc
  note: Q_dc
  note: dw_c
  note: w_c
  note: Q_c
  x_d : Inport
  dx_d : Inport  Port=2
  ddx_d : Inport  Port=3
  h : Inport  Port=4
  Demux : Demux  Outputs=[3,3]
  Demux1 : Demux  Outputs=[3, 4, 1]
  Demux2 : Demux  Outputs=[3,3,1]
  Demux3 : Demux  Outputs=[3,3,1]
  Gain : Gain  Gain=D_p  Multiplication=Matrix(K*u)  OutDataTypeStr=Inherit: Same as input  ParamDataTypeStr=Inherit: Same as input
  Gain1 : Gain  Gain=K_p  Multiplication=Matrix(K*u)  OutDataTypeStr=Inherit: Same as input  ParamDataTypeStr=Inherit: Same as input
  Gain2 : Gain  Gain=D_o  Multiplication=Matrix(K*u)  OutDataTypeStr=Inherit: Same as input  ParamDataTypeStr=Inherit: Same as input
  Integrator : Integrator  InitialCondition=[0 0 0]
  Integrator1 : Integrator  InitialCondition=[0 0 0]
  Integrator2 : Integrator  InitialCondition=[0 0 0]
  Integrator3 : Integrator  InitialCondition=[1 0 0 0]
  Matrix Gain2 : StateSpace  A=[]  B=[]  C=[]  D=K  X0=0  mask(Matrix Gain){K=inv(M_p)}
      mask prompts: K "Gain matrix:"
      mask help: Matrix Gain.
      mask Help: Multiplies input vector by entered matrix to produce output vector (y=Au).
      mask Display: disp('inv(Mp)')
  Matrix Gain3 : StateSpace  A=[]  B=[]  C=[]  D=K  X0=0  mask(Matrix Gain){K=inv(M_o)}
      mask prompts: K "Gain matrix:"
      mask help: Matrix Gain.
      mask Help: Multiplies input vector by entered matrix to produce output vector (y=Au).
      mask Display: disp('inv(Mo)')
  Mux : Mux  Inputs=3
  Mux1 : Mux  Inputs=3
  Mux2 : Mux  Inputs=[3,4,1]
  Subsystem : Subsystem
      mask Display: disp('2*tr(E)*Ko')
  Subsystem1 : Subsystem
      mask Display: disp('Quaternion\n Propagation')
  Subsystem2 : Subsystem
      mask Display: disp('Qproduct')
  Subsystem3 : Subsystem
  Subsystem4 : Subsystem
  Subsystem6 : Subsystem
  Subsystem7 : Subsystem
  Sum11 : Sum  Inputs=-+|  SaturateOnIntegerOverflow=on  InputSameDT=on  OutDataTypeStr=Inherit: Same as first input
  Sum2 : Sum  Inputs=|++  SaturateOnIntegerOverflow=on  InputSameDT=on  OutDataTypeStr=Inherit: Same as first input
  Sum3 : Sum  Inputs=|++  SaturateOnIntegerOverflow=on  InputSameDT=on  OutDataTypeStr=Inherit: Same as first input
  Sum4 : Sum  Inputs=-+|  SaturateOnIntegerOverflow=on  InputSameDT=on  OutDataTypeStr=Inherit: Same as first input
  Sum5 : Sum  Inputs=|+-  SaturateOnIntegerOverflow=on  InputSameDT=on  OutDataTypeStr=Inherit: Same as first input
  Sum6 : Sum  Inputs=|+-  SaturateOnIntegerOverflow=on  InputSameDT=on  OutDataTypeStr=Inherit: Same as first input
  Sum7 : Sum  Inputs=++|  SaturateOnIntegerOverflow=on  InputSameDT=on  OutDataTypeStr=Inherit: Same as first input
  Sum8 : Sum  Inputs=++|  SaturateOnIntegerOverflow=on  InputSameDT=on  OutDataTypeStr=Inherit: Same as first input
  Sum9 : Sum  Inputs=++|  SaturateOnIntegerOverflow=on  InputSameDT=on  OutDataTypeStr=Inherit: Same as first input
  x_c : Outport
  dx_c : Outport  Port=2
  ddx_c : Outport  Port=3
  wires:
  Demux1/2 -> Subsystem2/2(Q_1)
  Subsystem2/1(Out1) -> Mux2/2
  Mux2/1 -> x_c/1
  Demux3/2 -> Sum3/2
  Demux3/3 -> Mux/3
  Mux1/1 -> dx_c/1
  Demux1/3 -> Mux2/3
  Demux2/3 -> Mux1/3
  Gain1/1 -> Sum5/2
  Gain/1 -> Sum6/2
  Subsystem1/1(Out1) -> Subsystem6/1(In1)
  Subsystem/1(Out1) -> Sum4/1
  Sum8/1 -> Mux1/1
  Sum6/1 -> Matrix Gain2/1
  Integrator1/1 -> Sum7/2, Gain1/1
  Sum5/1 -> Sum6/1
  Integrator/1 -> Subsystem7/1(In1)
  Integrator2/1 -> Subsystem1/2(w_dc), Gain2/1, Sum2/1
  Matrix Gain3/1 -> Subsystem4/1(In1)
  Sum2/1 -> Mux1/2
  h/1 -> Demux/1
  Sum9/1 -> Mux/1
  Mux/1 -> ddx_c/1
  Gain2/1 -> Sum11/1
  Sum11/1 -> Matrix Gain3/1
  Sum4/1 -> Sum11/2
  x_d/1 -> Demux1/1
  dx_d/1 -> Demux2/1
  ddx_d/1 -> Demux3/1
  Demux1/1 -> Sum7/1
  Demux2/2 -> Sum2/2
  Demux2/1 -> Sum8/1
  Demux3/1 -> Sum9/1
  Sum3/1 -> Mux/2
  Integrator3/1 -> Subsystem2/1(Q_2), Subsystem/1(In1), Subsystem1/1(Q_dc)
  Sum7/1 -> Mux2/1
  Demux/1 -> Sum5/1
  Demux/2 -> Sum4/2
  Subsystem3/1(Out1) -> Integrator/1, Sum9/2
  Matrix Gain2/1 -> Subsystem3/1(In1)
  Subsystem6/1(Out1) -> Integrator3/1
  Subsystem7/1(Out1) -> Sum8/2, Gain/1, Integrator1/1
  Subsystem4/1(Out1) -> Sum3/1, Integrator2/1

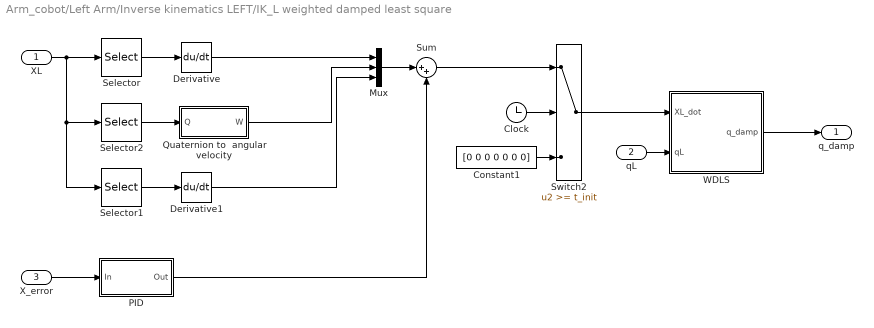
== system Arm_cobot/Left Arm/Inverse kinematics LEFT/IK_L weighted damped least square ==
  XL : Inport
  qL : Inport  Port=2
  X_error : Inport  Port=3
  Clock : Clock
  Constant1 : Constant  Value=[0 0 0 0 0 0 0]
  Derivative : Derivative
  Derivative1 : Derivative
  Mux : Mux  Inputs=3
  PID : Subsystem
  Quaternion to  angular velocity : Subsystem
  Selector : Selector  InputPortWidth=8  Indices=[1:3]
  Selector1 : Selector  InputPortWidth=8  Indices=[8]
  Selector2 : Selector  InputPortWidth=8  Indices=[4:7]
  Sum : Sum  Inputs=|++
  Switch2 : Switch  Threshold=t_init  SaturateOnIntegerOverflow=on  InputSameDT=on
  WDLS : Subsystem
  q_damp : Outport
  wires:
  Derivative1/1 -> Mux/3
  Derivative/1 -> Mux/1
  Selector2/1 -> Quaternion to  angular velocity/1(Q)
  Selector/1 -> Derivative/1
  Switch2/1 -> WDLS/1(XL_dot)
  Quaternion to  angular velocity/1(W) -> Mux/2
  XL/1 -> Selector/1, Selector2/1, Selector1/1
  qL/1 -> WDLS/2(qL)
  WDLS/1(q_damp) -> q_damp/1
  Constant1/1 -> Switch2/3
  Clock/1 -> Switch2/2
  Selector1/1 -> Derivative1/1
  X_error/1 -> PID/1(In)
  Mux/1 -> Sum/1
  Sum/1 -> Switch2/1
  PID/1(Out) -> Sum/2

== system Arm_cobot/Left Arm/Inverse kinematics LEFT/pose error in task space ==
  x_d : Inport
  x_m : Inport  Port=2
  qL : Inport  Port=3
  Embedded MATLAB Function : MATLAB Function  TreatAsAtomicUnit=on
  Mux1 : Mux  Inputs=2
  S-Function : S-Function  FunctionName=PoseError_S  EnableBusSupport=off
  X_error : Outport
  wires:
  Mux1/1 -> S-Function/1
  x_m/1 -> Mux1/2
  x_d/1 -> Mux1/1
  S-Function/1 -> Embedded MATLAB Function/1(errIn)
  Embedded MATLAB Function/1(errOut) -> X_error/1
  qL/1 -> Embedded MATLAB Function/2(qIn)

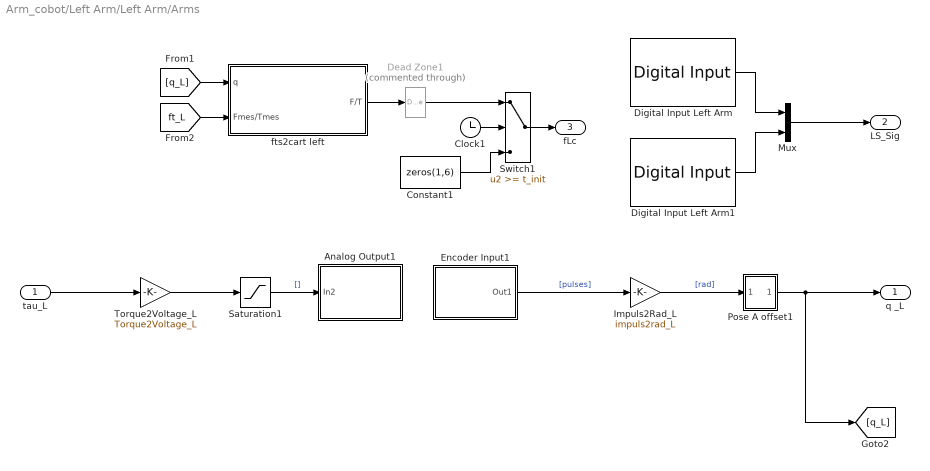
== system Arm_cobot/Left Arm/Left Arm/Arms ==
  tau_L : Inport
  Analog Output1 : Subsystem
      mask Display: disp('DAC')
  Clock1 : Clock
  Constant1 : Constant  Value=zeros(1,6)
  Dead Zone1 : DeadZone  Commented=through  LowerValue=[-2.5 -2.5 -2.5 -0.25 -0.25 -0.25]  UpperValue=[2.5 2.5 2.5 0.25 0.25 0.25]  SaturateOnIntegerOverflow=on
  Digital Input Left Arm : sensoray/Digital Input  BoardNumber=2  Channels=[35 34 33 32]  SampleTime=simget(bdroot,'FixedStep')
  Digital Input Left Arm1 : sensoray/Digital Input  BoardNumber=3  Channels=[35 34 33]  SampleTime=simget(bdroot,'FixedStep')
  Encoder Input1 : Subsystem
      mask Display: disp('ENC')
  Impuls2Rad_L : Gain  Gain=impuls2rad_L  SaturateOnIntegerOverflow=on  OutDataTypeStr=Inherit: Same as input  ParamDataTypeStr=Inherit: Same as input
  Mux : Mux  Inputs=2
  Pose A offset1 : Subsystem
      mask Display: disp('Pose\nOffset')
  Saturation1 : Saturate  UpperLimit=umaxL  LowerLimit=uminL
  Switch1 : Switch  Threshold=t_init  SaturateOnIntegerOverflow=on  InputSameDT=on
  Torque2Voltage_L : Gain  Gain=Torque2Voltage_L  SaturateOnIntegerOverflow=on  OutDataTypeStr=Inherit: Same as input  ParamDataTypeStr=Inherit: Same as input
  fts2cart left : Subsystem  mask(Transformation of measured force/torque of FT-sensor into the Newtonian frame){MEE=mEE_L, LEE=d_FTS_EE_L, OFFbee=p_EE_o_L, Fcal=Fcal_L, Tcal=Tcal_L, LTCP=LTool_L}
      mask prompts: MEE "Endeffector mass"; LEE "Distance of endeffector to FT-sensor coordinate system"; OFFbee "Location of center of gravity of the endeffector in endeffector coordinate system"; Fcal "Force acting at the FT-sensor  in the moment of calibration, given in FTS coordinate system"; Tcal "Torque acting at the FT-sensor in the moment of calibration given in the FTS coordinate system"; LTCP "Location of tool center point (point at which the master motion will be mapped) given in the FT-sensor coordinate system"
      mask help: Transforms the measured force/torque given in the FT-sensor coordinate system into the Newtonian frame. Additionally the endeffector mass and inertia are compensated.
  q _L : Outport
  LS_Sig : Outport  Port=2
  fLc : Outport  Port=3
  wires:
  Pose A offset1/1(out) -> q _L/1, [q_L]
  Encoder Input1/1(Out1) -> Impuls2Rad_L/1  "[pulses]"
  Impuls2Rad_L/1 -> Pose A offset1/1(in)  "[rad]"
  Saturation1/1 -> Analog Output1/1(In2)  "[]"
  Torque2Voltage_L/1 -> Saturation1/1
  fts2cart left/1(F/T) -> Dead Zone1/1
  [q_L] -> fts2cart left/1(q)
  Dead Zone1/1 -> Switch1/1
  Switch1/1 -> fLc/1
  Clock1/1 -> Switch1/2
  Constant1/1 -> Switch1/3
  Mux/1 -> LS_Sig/1
  Digital Input Left Arm/1 -> Mux/1
  Digital Input Left Arm1/1 -> Mux/2
  tau_L/1 -> Torque2Voltage_L/1
  [ft_L] -> fts2cart left/2(Fmes/Tmes)
